simulink model "robosim"  (Simulink 7.5)
settings: Solver=ode45  StartTime=0.0  StopTime=10  RelTol=1e-6
values from neighbouring files (symbols this model uses):
  F = zeros(ny*nP,nx+nu)    [gpc.m]    (also in questao2.m = [-K,zeros(1,2);zeros(1,2) -K])
libraries: simulink x1
settings Model: Creator=DH55PJ02  LastModifiedBy=DH55PJ02
settings OptimizationCC: InlineInvariantSignals=on
settings DebuggingCC: SaveWithParameterizedLinksMsg=none  SignalResolutionControl=TryResolveAllWithWarning  SolverPrmCheckMsg=none  MultiTaskCondExecSysMsg=none  StrictBusMsg=Warning
settings HardwareCC: TargetUnknown=on
settings RTWCC: IncludeERTFirstTime=on
settings GRTTargetCC: TargetFcnLib=ansi_tfl_tmw.mat

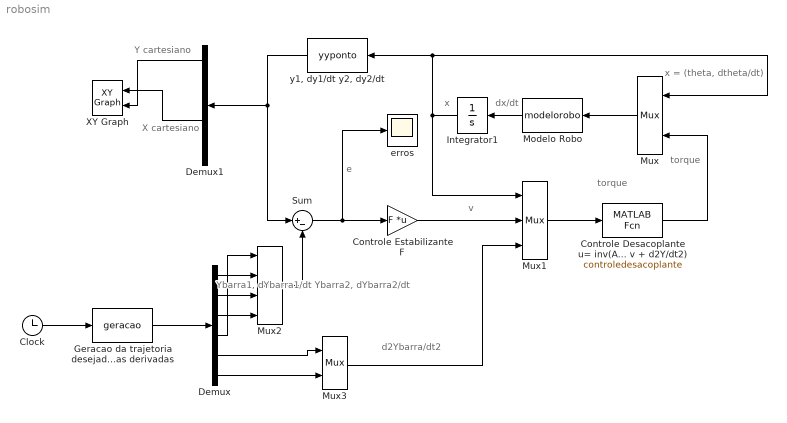
== system robosim ==
  note: x
  note: dx/dt
  note: torque
  note: Ybarra1, dYbarra1/dt
      |                               Ybarra2, dYbarra2/dt
  note: v
  note: d2Ybarra/dt2
  note: e
  note: torque
  note: x = (theta, dtheta/dt)
  note: Y cartesiano
  note: X cartesiano
  Clock : Clock
      settings: Decimation=10
  Controle Desacoplante u= inv(A) (-a + v + d2Y/dt2) : MATLABFcn  MATLABFcn=controledesacoplante  OutputDimensions=2
  Controle Estabilizante F : Gain  Gain=F  Multiplication=Matrix(K*u)  ParameterDataType=sfix(16)  ParameterScaling=2^0  OutDataType=sfix(16)  OutScaling=2^0
  Demux : Demux  Outputs=6
  Demux1 : Demux
  Geracao da trajetoria desejada Ybarra(t) e  suas derivadas : MATLABFcn  MATLABFcn=geracao  OutputDimensions=6
  Integrator1 : Integrator  InitialCondition=[0 pi/4 0 0]
  Modelo Robo : MATLABFcn  MATLABFcn=modelorobo  OutputDimensions=4
  Mux : Mux  Inputs=2
  Mux1 : Mux  Inputs=3
  Mux2 : Mux
  Mux3 : Mux  Inputs=2
  Sum : Sum  Inputs=|+-  OutDataType=sfix(16)  OutScaling=2^0
  XY Graph : simulink/Sinks/XY Graph  SystemSampleTime=-1  xmin=-2  xmax=2  ymin=-2  ymax=2  st=-1
  erros : Scope
  "y1, dy1/dt y2, dy2/dt" : MATLABFcn  MATLABFcn=yyponto  OutputDimensions=4
  wires:
  Modelo Robo/1 -> Integrator1/1
  Mux/1 -> Modelo Robo/1
  Integrator1/1 -> "y1, dy1/dt y2, dy2/dt"/1, Mux/1, Mux1/1
  Controle Desacoplante u= inv(A) (-a + v + d2Y/dt2)/1 -> Mux/2
  Geracao da trajetoria desejada Ybarra(t) e  suas derivadas/1 -> Demux/1
  Mux1/1 -> Controle Desacoplante u= inv(A) (-a + v + d2Y/dt2)/1
  Sum/1 -> Controle Estabilizante F/1, erros/1
  Clock/1 -> Geracao da trajetoria desejada Ybarra(t) e  suas derivadas/1
  "y1, dy1/dt y2, dy2/dt"/1 -> Sum/1, Demux1/1
  Demux/1 -> Mux2/1
  Demux/2 -> Mux2/2
  Demux/3 -> Mux2/3
  Demux/4 -> Mux2/4
  Mux2/1 -> Sum/2
  Demux/5 -> Mux3/1
  Demux/6 -> Mux3/2
  Controle Estabilizante F/1 -> Mux1/2
  Mux3/1 -> Mux1/3
  Demux1/3 -> XY Graph/1
  Demux1/1 -> XY Graph/2
